simulink model "ETB_NLDC"  (R2024b)
settings: Solver=ode1  StartTime=0.0  StopTime=5  FixedStep=1e-5  MaxStep=0.001  RelTol=0.001
undefined symbols (not defined in the file): K, K_r, sigbuilder_block
settings Model: Creator=paolo  LastModifiedBy=lowan
settings SolverCC: AlgebraicLoopSolver=TrustRegion
settings DebuggingCC: ArithmeticOperatorsInVariantConditions=warning
settings SFSimCC: CustomCodeUndefinedFunction=UseInterfaceOnly
settings RTWCC: GPUComputeCapability=3.5  DLArmComputeVersion=19.05

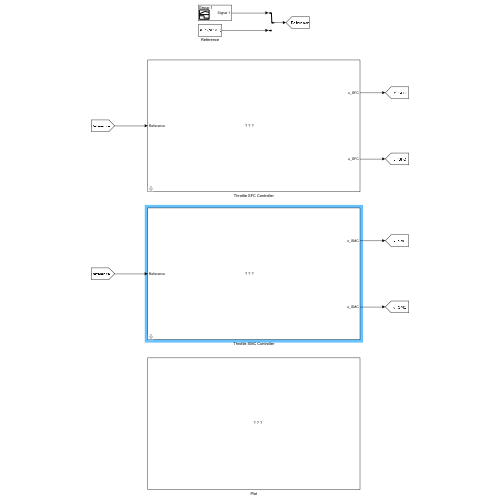
[thumbnail: Simulink's stored preview of the top-level diagram]
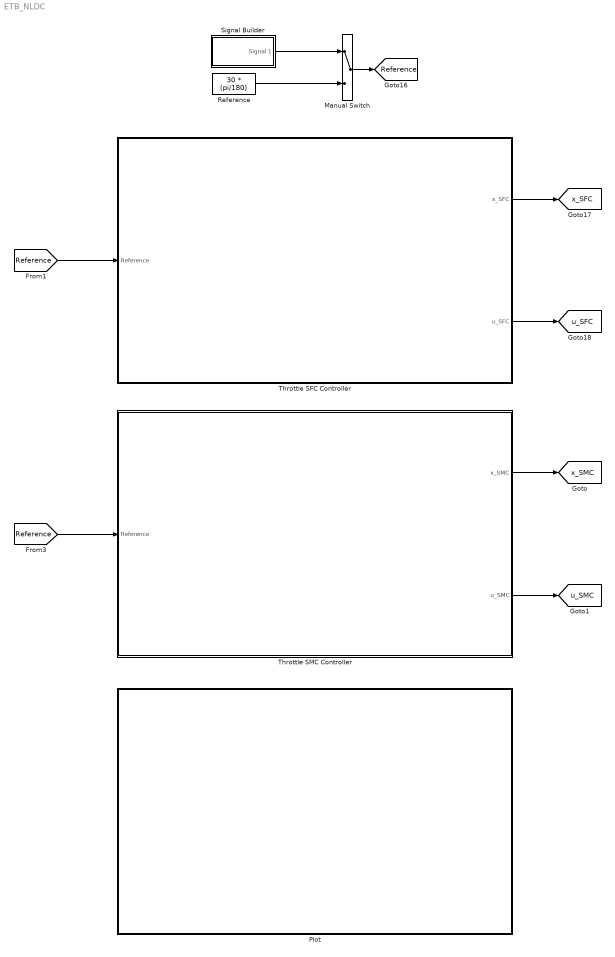
== system ETB_NLDC ==
  Manual Switch : ManualSwitch
  Plot : Subsystem
      mask Display: image('PlotIcon.png'); % Use "Edit Image" on toolstrip to change.
  Reference : Constant  Value=30 * (pi/180)
  Signal Builder : Subsystem  Tag=STV Subsys  LoadFcn=sigbuilder_block('load');  StartFcn=sigbuilder_block('start');  StopFcn=sigbuilder_block('stop');  ClipboardFcn=sigbuilder_block('clipboard');  mask(Sigbuilder block){tuvar=[0:10]}
      mask help: Simulink:masks:SigbuilderBlock_MD
      mask init:
      | if ~strcmp(get_param(bdroot(gcbh),'SimulationStatus'),'stopped') tuvar = sigbuilder_block('maskInit'); end
      settings: CopyFcn=sigbuilder_block('copy');  DeleteFcn=sigbuilder_block('delete');  ModelCloseFcn=sigbuilder_block('modelClose');  PreSaveFcn=sigbuilder_block('preSave');  PauseFcn=sigbuilder_block('pause');  ContinueFcn=sigbuilder_block('continue');  NameChangeFcn=sigbuilder_block('namechange');  OpenFcn=sigbuilder_block('open',[2326.2 204 550.2 399.6 ]);  CloseFcn=sigbuilder_block('close');
      mask Display: plot(0, 0, 100, 100,[2, 2, 32, 32, 2], [68, 8, 8, 68, 68],[32, 2], [38, 38], [32, 19, 2],[53, 60, 44], [32, 17, 17, 2],[16, 16, 31, 31]);txt = getActiveGroup(gcbh);text(2, 100, txt,'verticalAlignment', 'top');
  Throttle SFC Controller : Subsystem  mask{dist_switch=off, Amp_disturbance=3, Freq_disturbance=10, unc_switch=off, unc=1.3}
      mask prompts: dist_switch "Enable Disturbance"; Amp_disturbance "Amplitude of Disturb"; Freq_disturbance "Frequency of Disturb"; unc_switch "Enable Uncertainity"; unc "Uncertainity Value"
      mask DialogControl ParameterGroupVar Prompt: Disturbance Parameter
      mask DialogControl Container3 Prompt: Uncertainity Parameter
      mask Display: image('ThrottleBody_SFC.png'); % Use "Edit Image" on toolstrip to change.
  Throttle SMC Controller : Subsystem  mask{dist_switch=off, Amp_disturbance=3, Freq_disturbance=10, unc_switch=off, unc=1.3}
      mask prompts: dist_switch "Enable Disturbance"; Amp_disturbance "Amplitude of Disturb"; Freq_disturbance "Frequency of Disturb"; unc_switch "Enable Uncertainity"; unc "Uncertainity Value"
      mask DialogControl ParameterGroupVar Prompt: Disturbance Parameter
      mask DialogControl Container3 Prompt: Uncertainity Parameter
      mask Display: image('ThrottleBody_SMC.png'); % Use "Edit Image" on toolstrip to change.
  tag scope: Reference=global, u_SFC=global, u_SMC=global, x_SFC=global, x_SMC=global
  wires:
  Throttle SFC Controller/1(x_SFC) -> [x_SFC]
  Throttle SFC Controller/2(u_SFC) -> [u_SFC]
  Signal Builder/1(Signal 1) -> Manual Switch/1
  Reference/1 -> Manual Switch/2
  Manual Switch/1 -> [Reference]
  Throttle SMC Controller/1(x_SMC) -> [x_SMC]
  Throttle SMC Controller/2(u_SMC) -> [u_SMC]
  [Reference] -> Throttle SFC Controller/1(Reference)
  [Reference] -> Throttle SMC Controller/1(Reference)

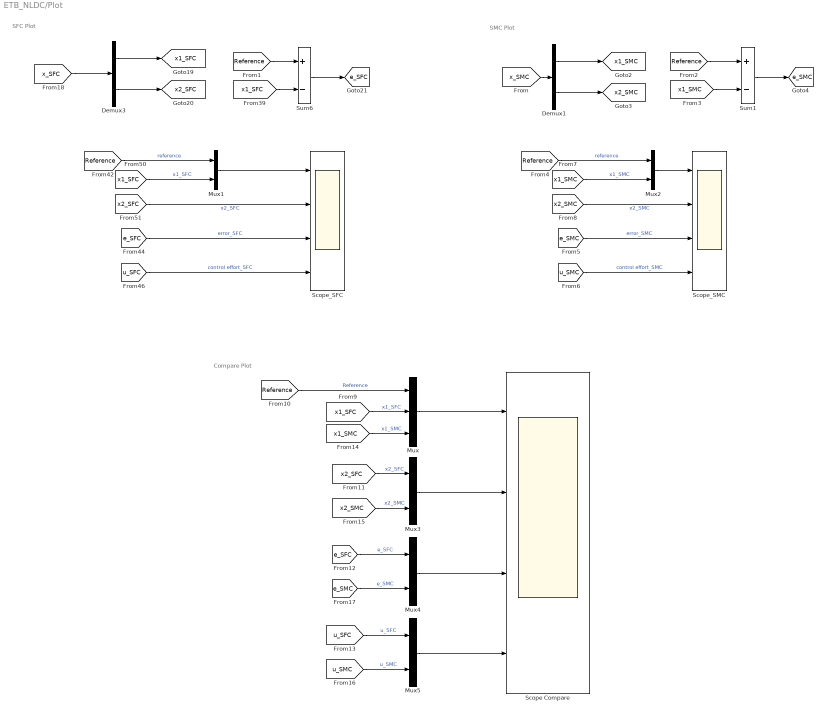
== system ETB_NLDC/Plot ==
  note: Compare Plot
  note: SMC Plot
  note: SFC Plot
  Demux1 : Demux  Outputs=2
  Demux3 : Demux  Outputs=2
  Mux : Mux  Inputs=3
  Mux{1..5} (5 alike) : Mux  Inputs=2
  Scope Compare : Scope  NumInputPorts=4
  Scope_SFC : Scope  NumInputPorts=4
  Scope_SMC : Scope  NumInputPorts=4
  Sum1 : Sum  Inputs=+-
  Sum6 : Sum  Inputs=+-
  tag scope: e_SFC=global, e_SMC=global, x1_SFC=global, x1_SMC=global, x2_SFC=global, x2_SMC=global
  wires:
  [x1_SFC] -> Mux1/2  "x1_SFC"
  [x2_SFC] -> Scope_SFC/2  "x2_SFC"
  Demux3/2 -> [x2_SFC]
  [x1_SFC] -> Sum6/2
  [e_SFC] -> Scope_SFC/3  "error_SFC"
  Sum6/1 -> [e_SFC]
  [Reference] -> Mux1/1  "reference"
  [u_SFC] -> Scope_SFC/4  "control effort_SFC"
  Demux3/1 -> [x1_SFC]
  Mux1/1 -> Scope_SFC/1
  [Reference] -> Sum6/1
  Demux1/1 -> [x1_SMC]
  Demux1/2 -> [x2_SMC]
  [Reference] -> Mux2/1  "reference"
  Mux2/1 -> Scope_SMC/1
  [x2_SMC] -> Scope_SMC/2  "x2_SMC"
  [Reference] -> Sum1/1
  [e_SMC] -> Scope_SMC/3  "error_SMC"
  [x1_SMC] -> Sum1/2
  [x1_SMC] -> Mux2/2  "x1_SMC"
  [u_SMC] -> Scope_SMC/4  "control effort_SMC"
  Sum1/1 -> [e_SMC]
  [Reference] -> Mux/1  "Reference"
  Mux3/1 -> Scope Compare/2
  Mux5/1 -> Scope Compare/4
  [x2_SFC] -> Mux3/1  "x2_SFC"
  [u_SMC] -> Mux5/2  "u_SMC"
  [u_SFC] -> Mux5/1  "u_SFC"
  Mux/1 -> Scope Compare/1
  [e_SFC] -> Mux4/1  "e_SFC"
  [x2_SMC] -> Mux3/2  "x2_SMC"
  [x1_SFC] -> Mux/2  "x1_SFC"
  [e_SMC] -> Mux4/2  "e_SMC"
  Mux4/1 -> Scope Compare/3
  [x1_SMC] -> Mux/3  "x1_SMC"
  [x_SFC] -> Demux3/1
  [x_SMC] -> Demux1/1

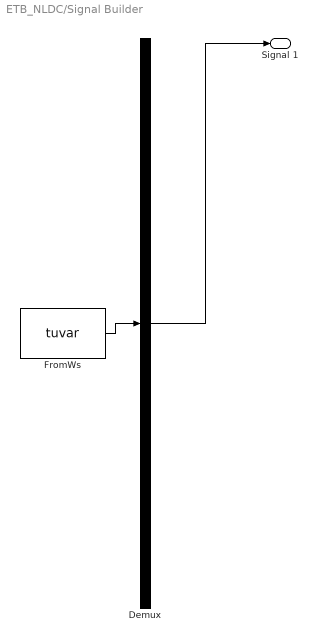
== system ETB_NLDC/Signal Builder ==
  Demux : Demux  Tag=STV Demux  Outputs=1
      settings: DisplayOption=none
  FromWs : FromWorkspace  Tag=STV FromWs  VariableName=tuvar
      SigBuilderData=|
      | common.afterFinalStr = 'Extrapolate'
      | common.sampleTime = 0
      | dataSet.timeRange = [0 10]
      | dataSet.name = 'Group 1'
      | sbobj.Groups.Name = 'Group 1'
      | sbobj.Groups.Signals.Name = 'Signal 1'
      | sbobj.Groups.Signals.XData = [0 2 4 4 6 6 10]
      | sbobj.Groups.Signals.YData = [0 1.3962634016 1.3962634016 1 1 0 0]
  Signal 1 : Outport  Tag=STV Outport
  wires:
  Demux/1 -> Signal 1/1
  FromWs/1 -> Demux/1

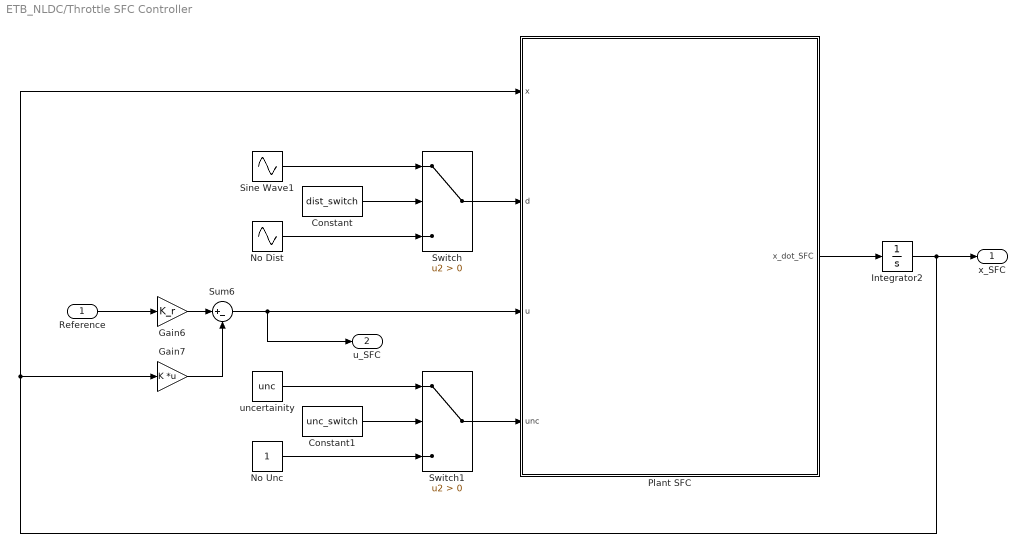
== system ETB_NLDC/Throttle SFC Controller ==
  Reference : Inport
  Constant : Constant  Value=dist_switch
  Constant1 : Constant  Value=unc_switch
  Gain6 : Gain  Gain=K_r
  Gain7 : Gain  Gain=K  Multiplication=Matrix(K*u)
  Integrator2 : Integrator
  No Dist : Sin  Amplitude=0  Frequency=0  SampleTime=0
  No Unc : Constant
  Plant SFC : MATLAB Function  TreatAsAtomicUnit=on
  Sine Wave1 : Sin  Amplitude=Amp_disturbance * (pi/180)  Frequency=Freq_disturbance  SampleTime=0
  Sum6 : Sum  Inputs=|+-
  Switch : Switch  Criteria=u2 > Threshold  SaturateOnIntegerOverflow=off  InputSameDT=off
  Switch1 : Switch  Criteria=u2 > Threshold  SaturateOnIntegerOverflow=off  InputSameDT=off
  uncertainity : Constant  Value=unc
  x_SFC : Outport
  u_SFC : Outport  Port=2
  wires:
  Sum6/1 -> u_SFC/1, Plant SFC/3(u)
  Gain6/1 -> Sum6/1
  Reference/1 -> Gain6/1
  Gain7/1 -> Sum6/2
  Plant SFC/1(x_dot_SFC) -> Integrator2/1
  Integrator2/1 -> Plant SFC/1(x), Gain7/1, x_SFC/1
  Constant/1 -> Switch/2
  Sine Wave1/1 -> Switch/1
  No Dist/1 -> Switch/3
  Switch/1 -> Plant SFC/2(d)
  No Unc/1 -> Switch1/3
  uncertainity/1 -> Switch1/1
  Constant1/1 -> Switch1/2
  Switch1/1 -> Plant SFC/4(unc)

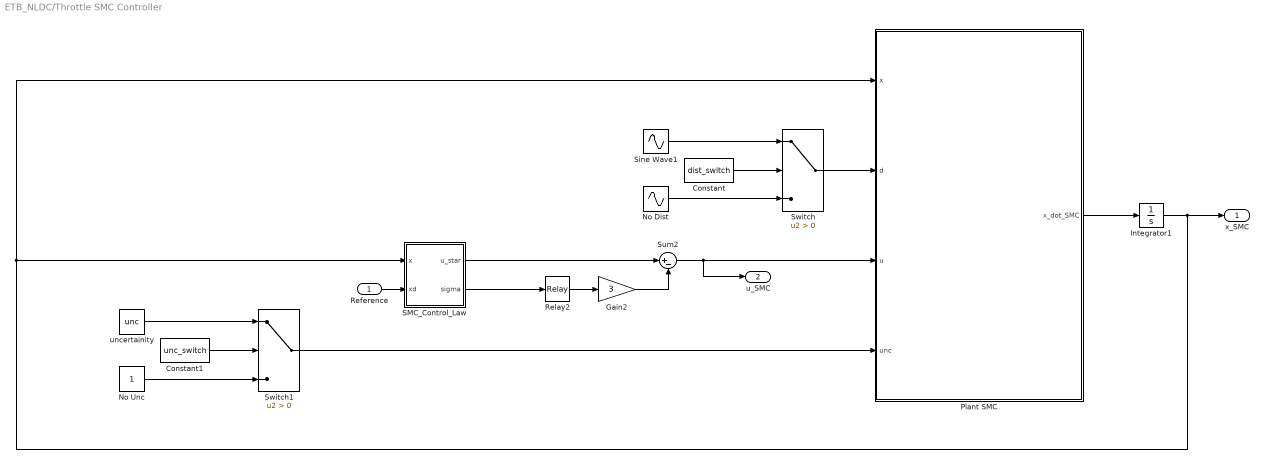
== system ETB_NLDC/Throttle SMC Controller ==
  Reference : Inport
  Constant : Constant  Value=dist_switch
  Constant1 : Constant  Value=unc_switch
  Gain2 : Gain  Gain=3
  Integrator1 : Integrator
  No Dist : Sin  Amplitude=0  Frequency=0  SampleTime=0
  No Unc : Constant
  Plant SMC : MATLAB Function  TreatAsAtomicUnit=on
  Relay2 : Relay  OnSwitchValue=0.01  OffSwitchValue=-0.01  OffOutputValue=-1
  SMC_Control_Law : MATLAB Function  TreatAsAtomicUnit=on
  Sine Wave1 : Sin  Amplitude=Amp_disturbance * (pi/180)  Frequency=Freq_disturbance  SampleTime=0
  Sum2 : Sum  Inputs=|+-
  Switch : Switch  Criteria=u2 > Threshold  SaturateOnIntegerOverflow=off  InputSameDT=off
  Switch1 : Switch  Criteria=u2 > Threshold  SaturateOnIntegerOverflow=off  InputSameDT=off
  uncertainity : Constant  Value=unc
  x_SMC : Outport
  u_SMC : Outport  Port=2
  wires:
  Reference/1 -> SMC_Control_Law/2(xd)
  Constant/1 -> Switch/2
  Sine Wave1/1 -> Switch/1
  No Dist/1 -> Switch/3
  No Unc/1 -> Switch1/3
  uncertainity/1 -> Switch1/1
  Constant1/1 -> Switch1/2
  Switch/1 -> Plant SMC/2(d)
  Integrator1/1 -> x_SMC/1, Plant SMC/1(x), SMC_Control_Law/1(x)
  Plant SMC/1(x_dot_SMC) -> Integrator1/1
  SMC_Control_Law/2(sigma) -> Relay2/1
  Relay2/1 -> Gain2/1
  Sum2/1 -> u_SMC/1, Plant SMC/3(u)
  Switch1/1 -> Plant SMC/4(unc)
  SMC_Control_Law/1(u_star) -> Sum2/1
  Gain2/1 -> Sum2/2

== matlab function ETB_NLDC/Throttle SMC Controller/SMC_Control_Law ==
  data: x input; u_star output; xd input; sigma output
function [u_star, sigma] = fcn(x,xd)
% Nominal Parameters
J  = 2.5e-4; 
k1 = 0.15;
k2 = 0.5;
b1 = 0.01;
b2 = 0.001;

x1 = x(1);
x2 = x(2);

% Sliding Surface Parameters
% p1 determines the convergence rate of the error
p1 = 20; 
p2 = 1;

% Sliding Surface Calculation
% sigma = p1 * error + p2 * error_dot (assuming xd_dot = 0)
sigma = p1*(x1 - xd) + p2*x2;

% Estimation of Resistive Torques
T_spring   = k1 * x1 + k2 * x1^3;         % Linear + Cubic Stiffness
T_friction = b1 * x2 + b2 * x2 * abs(x2); % Viscous + Aerodynamic Damping

% u_star computation:
% sigma_dot = p1*x2 + p2*x2_dot = 0
% p1*x2 + (p2/J) (u_star - T_spring - T_friction) = 0

u_star = T_spring + T_friction - (J * p1 / p2) * x2;
end

== matlab function ETB_NLDC/Throttle SMC Controller/Plant SMC ==
  data: x input size=2; d input; u input size=1; x_dot_SMC output size=2; unc input
function x_dot_SMC = Plant_SMC(x,d,u,unc)
% Parameters definition with Uncertainity injection
J  = 2.5e-4 * unc;
k1 = 0.15   * unc;
k2 = 0.5    * unc;
b1 = 0.01   * unc;
b2 = 0.001  * unc;

% System States
x1 = x(1); % Throttle Angle (theta) [rad]
x2 = x(2); % Angular Velocity (theta_dot) [rad/s]

% State Equation 1: Kinematics
x1_dot = x2;

% State Equation 2: Rotational Dynamics
% Balance of Moments: J * alpha = Torque_Motor + Disturbance - Stiffness - Damping
x2_dot = - (k1/J)*x1 - (k2/J)*x1^3 - (b1/J)*x2 - (b2/J)*x2*abs(x2) + (u + d)/J;

x_dot_SMC = [x1_dot; x2_dot];
end

== matlab function ETB_NLDC/Throttle SFC Controller/Plant SFC ==
  data: x input size=2; d input; u input size=1; x_dot_SFC output size=2; unc input
function x_dot_SFC = Plant_SFC(x,d,u,unc)
% Parameters definition with Uncertainity injection
J  = 2.5e-4 * unc;
k1 = 0.15   * unc;
k2 = 0.5    * unc;
b1 = 0.01   * unc;
b2 = 0.001  * unc;

% System States
x1 = x(1); % Throttle Angle (theta) [rad]
x2 = x(2); % Angular Velocity (theta_dot) [rad/s]

% State Equation 1: Kinematics
x1_dot = x2;

% State Equation 2: Rotational Dynamics
% Balance of Moments: J * alpha = Torque_Motor + Disturbance - Stiffness - Damping
x2_dot = - (k1/J)*x1 - (k2/J)*x1^3 - (b1/J)*x2 - (b2/J)*x2*abs(x2) + (u + d)/J;

x_dot_SFC = [x1_dot; x2_dot];
end
